simulink model "GhendyanoT2FMeioLinha1"  (R2021b)
settings: Solver=ode45  StartTime=0.0  StopTime=TempoSimulacao  RelTol=1e-3  EnableMultiTasking=on
values from neighbouring files (symbols this model uses):
  ccc1 = Ccc*d    [TesteRealCurtoFuses.m]    (also in TesteRealCurto_SemFuse.m)
  ccc2 = Ccc*d    [TesteRealCurtoFuses.m]    (also in TesteRealCurto_SemFuse.m)
  cct1 = Cct*d    [TesteRealCurtoFuses.m]    (also in TesteRealCurto_SemFuse.m)
  cct2 = Cct*d    [TesteRealCurtoFuses.m]    (also in TesteRealCurto_SemFuse.m)
  cequa1 = Ceq*d    [TesteRealCurtoFuses.m]    (also in TesteRealCurto_SemFuse.m)
  cequa2 = Ceq*d    [TesteRealCurtoFuses.m]    (also in TesteRealCurto_SemFuse.m)
  FatorSimulacao = 1e-3    (= 0.001)    [TesteRealCurtoFuses.m]    (also in TesteRealCurto_SemFuse.m)
  le = 1e-10    [TesteRealCurto.m]    (also in TesteRealCurtoFuses.m; TesteRealCurto_SemFuse.m)
  lm1 = lm    [TesteRealCurto.m]    (also in TesteRealCurtoFuses.m; TesteRealCurto_SemFuse.m)
  lm2 = lm    [TesteRealCurto.m]    (also in TesteRealCurtoFuses.m; TesteRealCurto_SemFuse.m)
  lp1 = lp    [TesteRealCurto.m]    (also in TesteRealCurtoFuses.m; TesteRealCurto_SemFuse.m)
  lp2 = lp    [TesteRealCurto.m]    (also in TesteRealCurtoFuses.m; TesteRealCurto_SemFuse.m)
  NRE = 1e-12    [TesteRealCurto.m]    (also in TesteRealCurtoFuses.m; TesteRealCurto_SemFuse.m)
  Raf1 = inf    [TesteRealCurto.m]    (also in TesteRealCurtoFuses.m; TesteRealCurto_SemFuse.m)
  Raf2 = inf    [TesteRealCurto.m]    (also in TesteRealCurtoFuses.m; TesteRealCurto_SemFuse.m)
  Rbf1 = inf    [TesteRealCurto.m]    (also in TesteRealCurtoFuses.m; TesteRealCurto_SemFuse.m)
  Rbf2 = inf    [TesteRealCurto.m]    (also in TesteRealCurtoFuses.m; TesteRealCurto_SemFuse.m)
  Rcf1 = inf    [TesteRealCurto.m]    (also in TesteRealCurtoFuses.m; TesteRealCurto_SemFuse.m)
  Rcf2 = inf    [TesteRealCurto.m]    (also in TesteRealCurtoFuses.m; TesteRealCurto_SemFuse.m)
  rm1 = rm    [TesteRealCurto.m]    (also in TesteRealCurtoFuses.m; TesteRealCurto_SemFuse.m)
  rm2 = rm    [TesteRealCurto.m]    (also in TesteRealCurtoFuses.m; TesteRealCurto_SemFuse.m)
  rp1 = rp    [TesteRealCurto.m]    (also in TesteRealCurtoFuses.m; TesteRealCurto_SemFuse.m)
  rp2 = rp    [TesteRealCurto.m]    (also in TesteRealCurtoFuses.m; TesteRealCurto_SemFuse.m)
  rtc1 = 8    [TesteRealCurto.m]    (also in TesteRealCurtoFuses.m; TesteRealCurto_SemFuse.m)
  rtc2 = 8    [TesteRealCurto.m]    (also in TesteRealCurtoFuses.m; TesteRealCurto_SemFuse.m)
  rti = 10    [TesteRealCurto.m]    (also in TesteRealCurtoFuses.m; TesteRealCurto_SemFuse.m)
undefined symbols (not defined in the file or in its folder): D11, Delta, m1
libraries: spsSeriesRLCBranchLib x26, spsRMSLib x14, spsBreakerLib x9, spsCurrentMeasurementLib x9, spsThreePhaseTransformerTwoWindingsLib x4, spsThreePhaseVIMeasurementLib x3, spsMutualInductanceLib x3, spsThreePhaseSeriesRLCLoadLib x2, spsThreePhaseSourceLib x1, spspowerguiLib x1
(part 2 of 2)

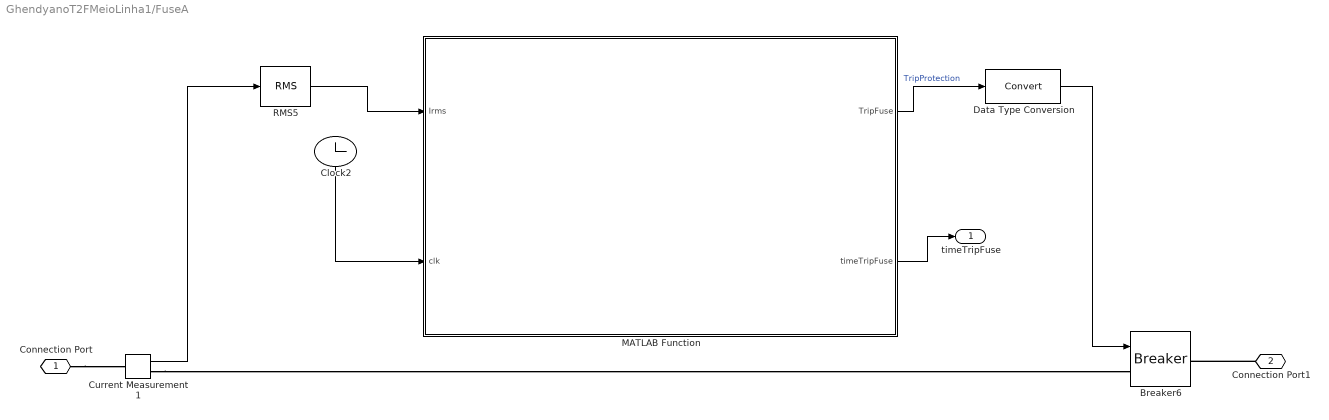
== system GhendyanoT2FMeioLinha1/FuseA ==
  Breaker6 : spsBreakerLib/Breaker  InitialState=1  SwitchingTimes="[1/60  5/60]"  External=on  BreakerResistance=0.01  SnubberResistance=1e6  SnubberCapacitance=inf  Measurements=None  MoreParameters=on  NoBreakLoop=off
      settings: SourceProductBaseCode=PS
  Clock2 : Clock
      settings: Decimation=1000
  Current Measurement1 : spsCurrentMeasurementLib/Current Measurement  PhasorSimulation=off  OutputType=Complex  PSBequivalent=0
  Data Type Conversion : DataTypeConversion
  MATLAB Function : MATLAB Function
  RMS5 : spsRMSLib/RMS  TrueRMS=on  Freq=60  RMSInit=0  Ts=0
  Connection Port : PMIOPort  Side=Right
  Connection Port1 : PMIOPort  Port=2  Side=Left
  timeTripFuse : Outport
  wires:
  MATLAB Function/1(TripFuse) -> Data Type Conversion/1  "TripProtection"
  RMS5/1 -> MATLAB Function/1(Irms)
  Data Type Conversion/1 -> Breaker6/1
  Current Measurement1/1 -> RMS5/1
  Clock2/1 -> MATLAB Function/2(clk)
  MATLAB Function/2(timeTripFuse) -> timeTripFuse/1
  connections:
  Current Measurement1/RConn1 -- Breaker6/LConn1
  Connection Port/RConn1 -- Current Measurement1/LConn1
  Connection Port1/RConn1 -- Breaker6/RConn1

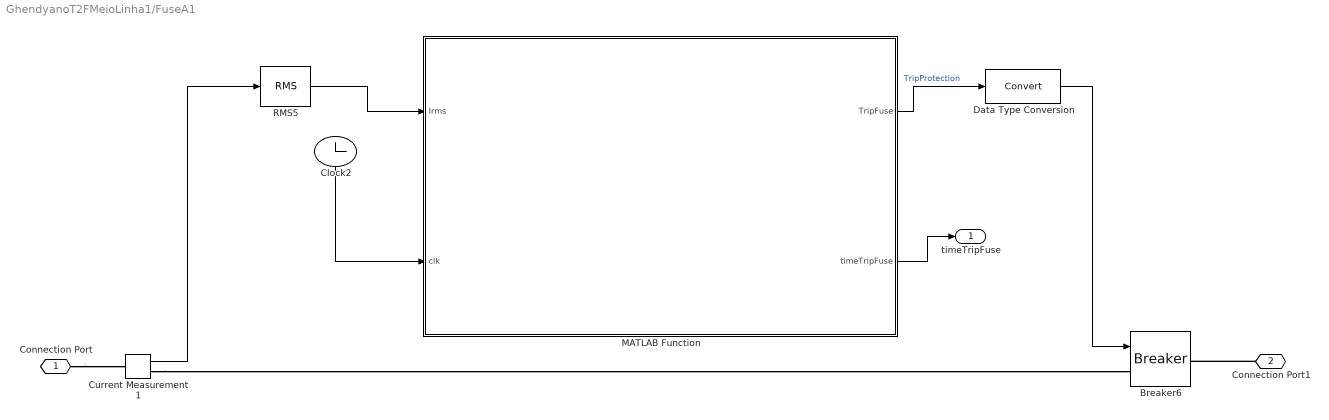
== system GhendyanoT2FMeioLinha1/FuseA1 ==
  Breaker6 : spsBreakerLib/Breaker  InitialState=1  SwitchingTimes="[1/60  5/60]"  External=on  BreakerResistance=0.01  SnubberResistance=1e6  SnubberCapacitance=inf  Measurements=None  MoreParameters=on  NoBreakLoop=off
      settings: SourceProductBaseCode=PS
  Clock2 : Clock
      settings: Decimation=1000
  Current Measurement1 : spsCurrentMeasurementLib/Current Measurement  PhasorSimulation=off  OutputType=Complex  PSBequivalent=0
  Data Type Conversion : DataTypeConversion
  MATLAB Function : MATLAB Function
  RMS5 : spsRMSLib/RMS  TrueRMS=on  Freq=60  RMSInit=0  Ts=0
  Connection Port : PMIOPort  Side=Right
  Connection Port1 : PMIOPort  Port=2  Side=Left
  timeTripFuse : Outport
  wires:
  MATLAB Function/1(TripFuse) -> Data Type Conversion/1  "TripProtection"
  RMS5/1 -> MATLAB Function/1(Irms)
  Data Type Conversion/1 -> Breaker6/1
  Current Measurement1/1 -> RMS5/1
  Clock2/1 -> MATLAB Function/2(clk)
  MATLAB Function/2(timeTripFuse) -> timeTripFuse/1
  connections:
  Current Measurement1/RConn1 -- Breaker6/LConn1
  Connection Port/RConn1 -- Current Measurement1/LConn1
  Connection Port1/RConn1 -- Breaker6/RConn1

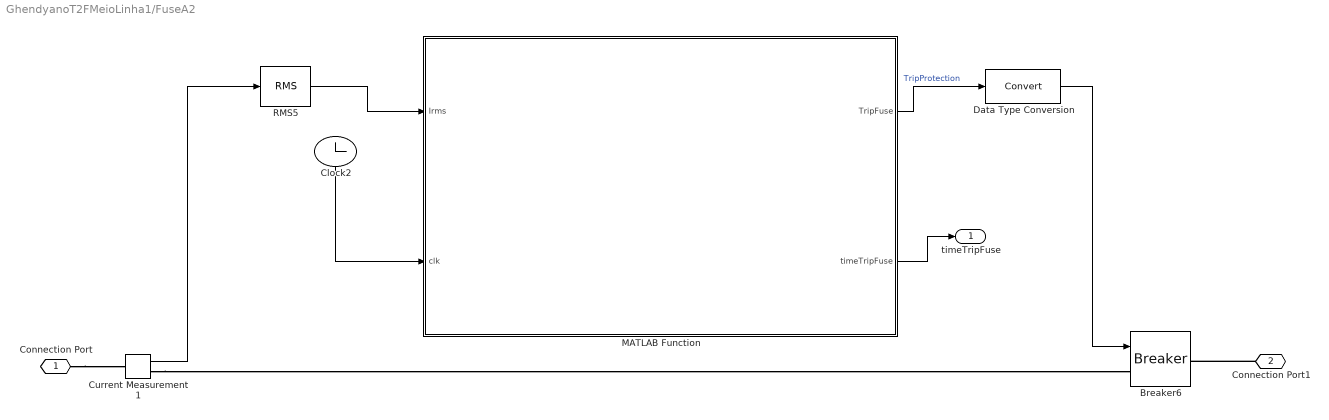
== system GhendyanoT2FMeioLinha1/FuseA2 ==
  Breaker6 : spsBreakerLib/Breaker  InitialState=1  SwitchingTimes="[1/60  5/60]"  External=on  BreakerResistance=0.01  SnubberResistance=1e6  SnubberCapacitance=inf  Measurements=None  MoreParameters=on  NoBreakLoop=off
      settings: SourceProductBaseCode=PS
  Clock2 : Clock
      settings: Decimation=1000
  Current Measurement1 : spsCurrentMeasurementLib/Current Measurement  PhasorSimulation=off  OutputType=Complex  PSBequivalent=0
  Data Type Conversion : DataTypeConversion
  MATLAB Function : MATLAB Function
  RMS5 : spsRMSLib/RMS  TrueRMS=on  Freq=60  RMSInit=0  Ts=0
  Connection Port : PMIOPort  Side=Right
  Connection Port1 : PMIOPort  Port=2  Side=Left
  timeTripFuse : Outport
  wires:
  MATLAB Function/1(TripFuse) -> Data Type Conversion/1  "TripProtection"
  RMS5/1 -> MATLAB Function/1(Irms)
  Data Type Conversion/1 -> Breaker6/1
  Current Measurement1/1 -> RMS5/1
  Clock2/1 -> MATLAB Function/2(clk)
  MATLAB Function/2(timeTripFuse) -> timeTripFuse/1
  connections:
  Current Measurement1/RConn1 -- Breaker6/LConn1
  Connection Port/RConn1 -- Current Measurement1/LConn1
  Connection Port1/RConn1 -- Breaker6/RConn1

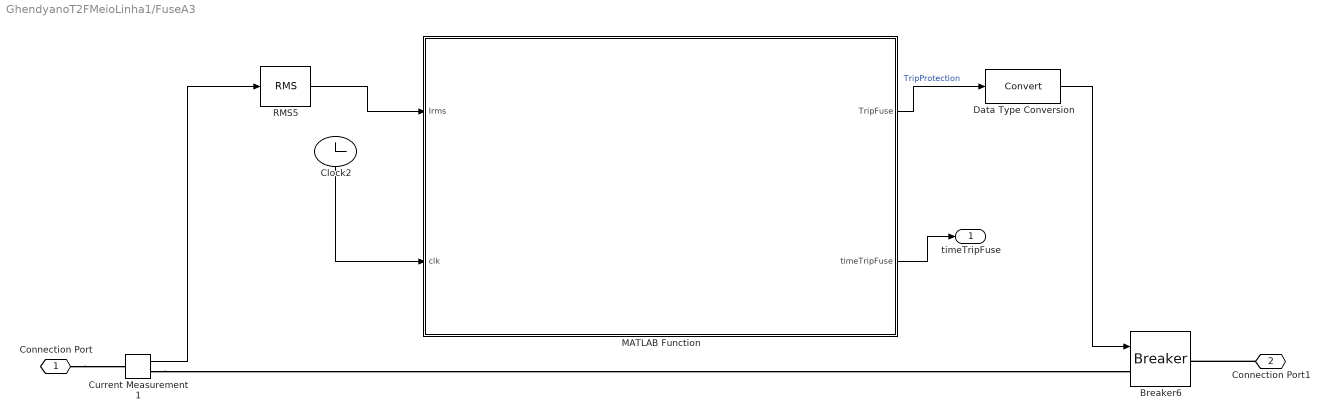
== system GhendyanoT2FMeioLinha1/FuseA3 ==
  Breaker6 : spsBreakerLib/Breaker  InitialState=1  SwitchingTimes="[1/60  5/60]"  External=on  BreakerResistance=0.01  SnubberResistance=1e6  SnubberCapacitance=inf  Measurements=None  MoreParameters=on  NoBreakLoop=off
      settings: SourceProductBaseCode=PS
  Clock2 : Clock
      settings: Decimation=1000
  Current Measurement1 : spsCurrentMeasurementLib/Current Measurement  PhasorSimulation=off  OutputType=Complex  PSBequivalent=0
  Data Type Conversion : DataTypeConversion
  MATLAB Function : MATLAB Function
  RMS5 : spsRMSLib/RMS  TrueRMS=on  Freq=60  RMSInit=0  Ts=0
  Connection Port : PMIOPort  Side=Right
  Connection Port1 : PMIOPort  Port=2  Side=Left
  timeTripFuse : Outport
  wires:
  MATLAB Function/1(TripFuse) -> Data Type Conversion/1  "TripProtection"
  RMS5/1 -> MATLAB Function/1(Irms)
  Data Type Conversion/1 -> Breaker6/1
  Current Measurement1/1 -> RMS5/1
  Clock2/1 -> MATLAB Function/2(clk)
  MATLAB Function/2(timeTripFuse) -> timeTripFuse/1
  connections:
  Current Measurement1/RConn1 -- Breaker6/LConn1
  Connection Port/RConn1 -- Current Measurement1/LConn1
  Connection Port1/RConn1 -- Breaker6/RConn1

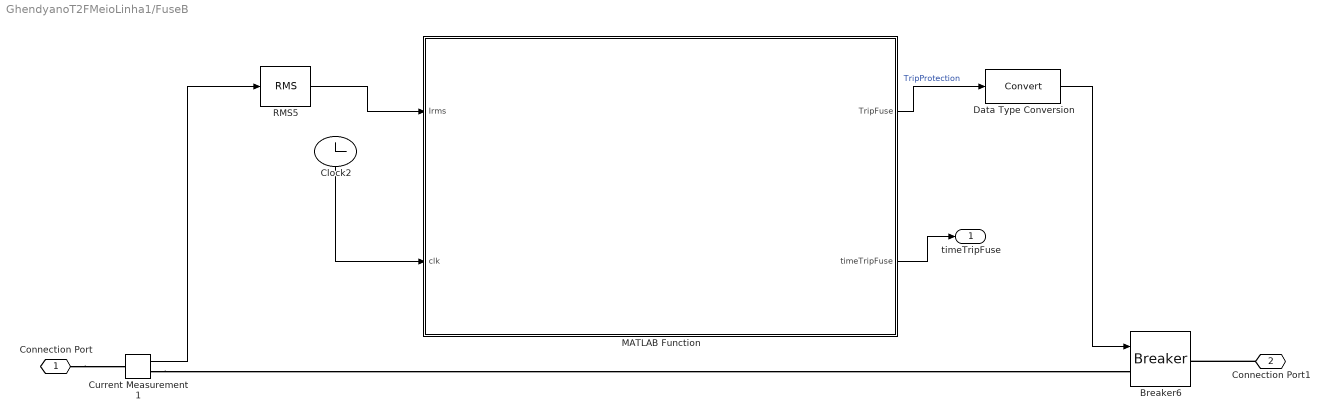
== system GhendyanoT2FMeioLinha1/FuseB ==
  Breaker6 : spsBreakerLib/Breaker  InitialState=1  SwitchingTimes="[1/60  5/60]"  External=on  BreakerResistance=0.01  SnubberResistance=1e6  SnubberCapacitance=inf  Measurements=None  MoreParameters=on  NoBreakLoop=off
      settings: SourceProductBaseCode=PS
  Clock2 : Clock
      settings: Decimation=1000
  Current Measurement1 : spsCurrentMeasurementLib/Current Measurement  PhasorSimulation=off  OutputType=Complex  PSBequivalent=0
  Data Type Conversion : DataTypeConversion
  MATLAB Function : MATLAB Function
  RMS5 : spsRMSLib/RMS  TrueRMS=on  Freq=60  RMSInit=0  Ts=0
  Connection Port : PMIOPort  Side=Right
  Connection Port1 : PMIOPort  Port=2  Side=Left
  timeTripFuse : Outport
  wires:
  MATLAB Function/1(TripFuse) -> Data Type Conversion/1  "TripProtection"
  RMS5/1 -> MATLAB Function/1(Irms)
  Data Type Conversion/1 -> Breaker6/1
  Current Measurement1/1 -> RMS5/1
  Clock2/1 -> MATLAB Function/2(clk)
  MATLAB Function/2(timeTripFuse) -> timeTripFuse/1
  connections:
  Current Measurement1/RConn1 -- Breaker6/LConn1
  Connection Port/RConn1 -- Current Measurement1/LConn1
  Connection Port1/RConn1 -- Breaker6/RConn1

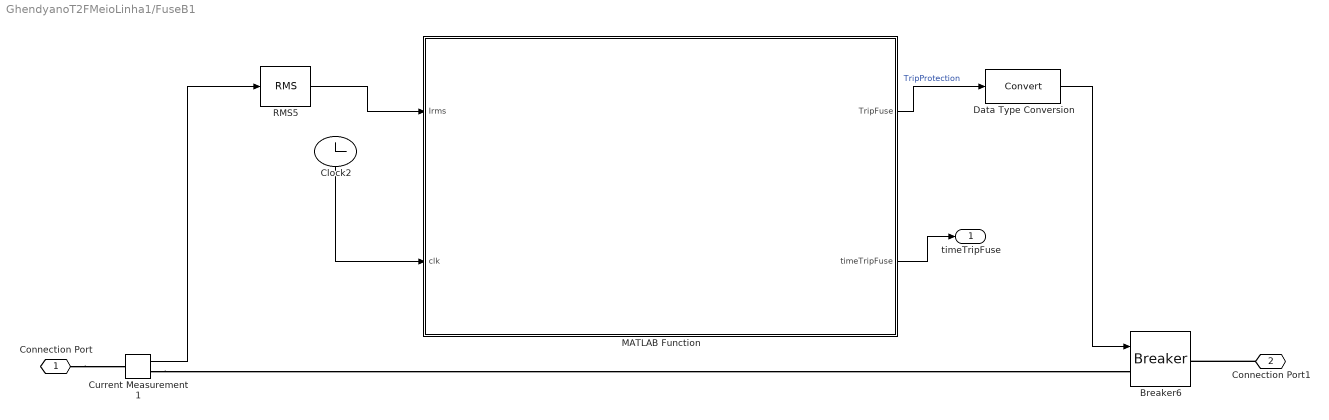
== system GhendyanoT2FMeioLinha1/FuseB1 ==
  Breaker6 : spsBreakerLib/Breaker  InitialState=1  SwitchingTimes="[1/60  5/60]"  External=on  BreakerResistance=0.01  SnubberResistance=1e6  SnubberCapacitance=inf  Measurements=None  MoreParameters=on  NoBreakLoop=off
      settings: SourceProductBaseCode=PS
  Clock2 : Clock
      settings: Decimation=1000
  Current Measurement1 : spsCurrentMeasurementLib/Current Measurement  PhasorSimulation=off  OutputType=Complex  PSBequivalent=0
  Data Type Conversion : DataTypeConversion
  MATLAB Function : MATLAB Function
  RMS5 : spsRMSLib/RMS  TrueRMS=on  Freq=60  RMSInit=0  Ts=0
  Connection Port : PMIOPort  Side=Right
  Connection Port1 : PMIOPort  Port=2  Side=Left
  timeTripFuse : Outport
  wires:
  MATLAB Function/1(TripFuse) -> Data Type Conversion/1  "TripProtection"
  RMS5/1 -> MATLAB Function/1(Irms)
  Data Type Conversion/1 -> Breaker6/1
  Current Measurement1/1 -> RMS5/1
  Clock2/1 -> MATLAB Function/2(clk)
  MATLAB Function/2(timeTripFuse) -> timeTripFuse/1
  connections:
  Current Measurement1/RConn1 -- Breaker6/LConn1
  Connection Port/RConn1 -- Current Measurement1/LConn1
  Connection Port1/RConn1 -- Breaker6/RConn1

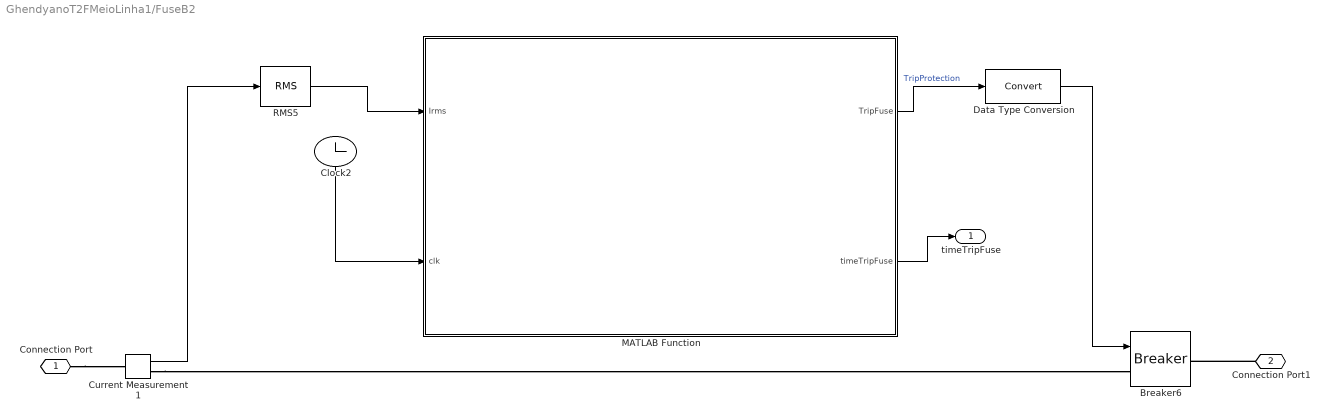
== system GhendyanoT2FMeioLinha1/FuseB2 ==
  Breaker6 : spsBreakerLib/Breaker  InitialState=1  SwitchingTimes="[1/60  5/60]"  External=on  BreakerResistance=0.01  SnubberResistance=1e6  SnubberCapacitance=inf  Measurements=None  MoreParameters=on  NoBreakLoop=off
      settings: SourceProductBaseCode=PS
  Clock2 : Clock
      settings: Decimation=1000
  Current Measurement1 : spsCurrentMeasurementLib/Current Measurement  PhasorSimulation=off  OutputType=Complex  PSBequivalent=0
  Data Type Conversion : DataTypeConversion
  MATLAB Function : MATLAB Function
  RMS5 : spsRMSLib/RMS  TrueRMS=on  Freq=60  RMSInit=0  Ts=0
  Connection Port : PMIOPort  Side=Right
  Connection Port1 : PMIOPort  Port=2  Side=Left
  timeTripFuse : Outport
  wires:
  MATLAB Function/1(TripFuse) -> Data Type Conversion/1  "TripProtection"
  RMS5/1 -> MATLAB Function/1(Irms)
  Data Type Conversion/1 -> Breaker6/1
  Current Measurement1/1 -> RMS5/1
  Clock2/1 -> MATLAB Function/2(clk)
  MATLAB Function/2(timeTripFuse) -> timeTripFuse/1
  connections:
  Current Measurement1/RConn1 -- Breaker6/LConn1
  Connection Port/RConn1 -- Current Measurement1/LConn1
  Connection Port1/RConn1 -- Breaker6/RConn1

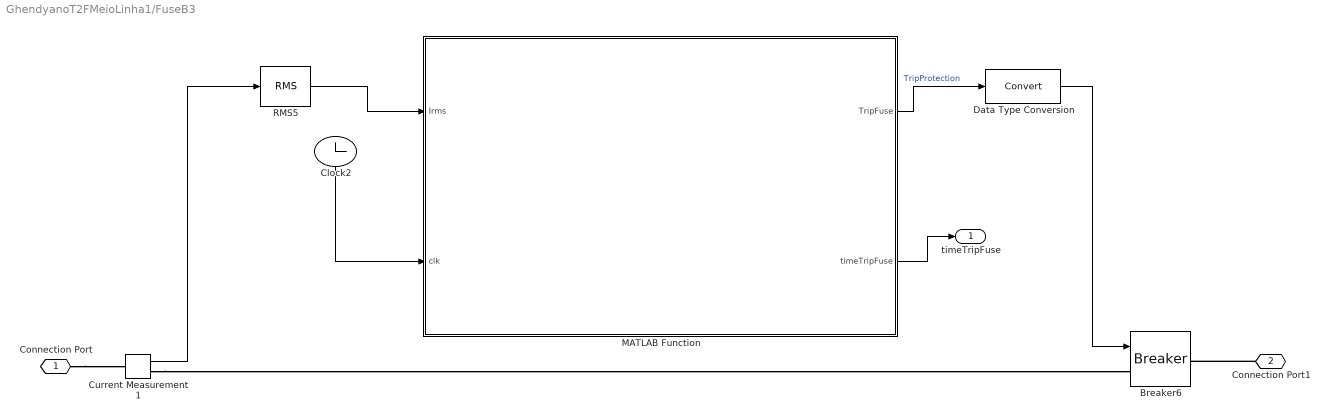
== system GhendyanoT2FMeioLinha1/FuseB3 ==
  Breaker6 : spsBreakerLib/Breaker  InitialState=1  SwitchingTimes="[1/60  5/60]"  External=on  BreakerResistance=0.01  SnubberResistance=1e6  SnubberCapacitance=inf  Measurements=None  MoreParameters=on  NoBreakLoop=off
      settings: SourceProductBaseCode=PS
  Clock2 : Clock
      settings: Decimation=1000
  Current Measurement1 : spsCurrentMeasurementLib/Current Measurement  PhasorSimulation=off  OutputType=Complex  PSBequivalent=0
  Data Type Conversion : DataTypeConversion
  MATLAB Function : MATLAB Function
  RMS5 : spsRMSLib/RMS  TrueRMS=on  Freq=60  RMSInit=0  Ts=0
  Connection Port : PMIOPort  Side=Right
  Connection Port1 : PMIOPort  Port=2  Side=Left
  timeTripFuse : Outport
  wires:
  MATLAB Function/1(TripFuse) -> Data Type Conversion/1  "TripProtection"
  RMS5/1 -> MATLAB Function/1(Irms)
  Data Type Conversion/1 -> Breaker6/1
  Current Measurement1/1 -> RMS5/1
  Clock2/1 -> MATLAB Function/2(clk)
  MATLAB Function/2(timeTripFuse) -> timeTripFuse/1
  connections:
  Current Measurement1/RConn1 -- Breaker6/LConn1
  Connection Port/RConn1 -- Current Measurement1/LConn1
  Connection Port1/RConn1 -- Breaker6/RConn1

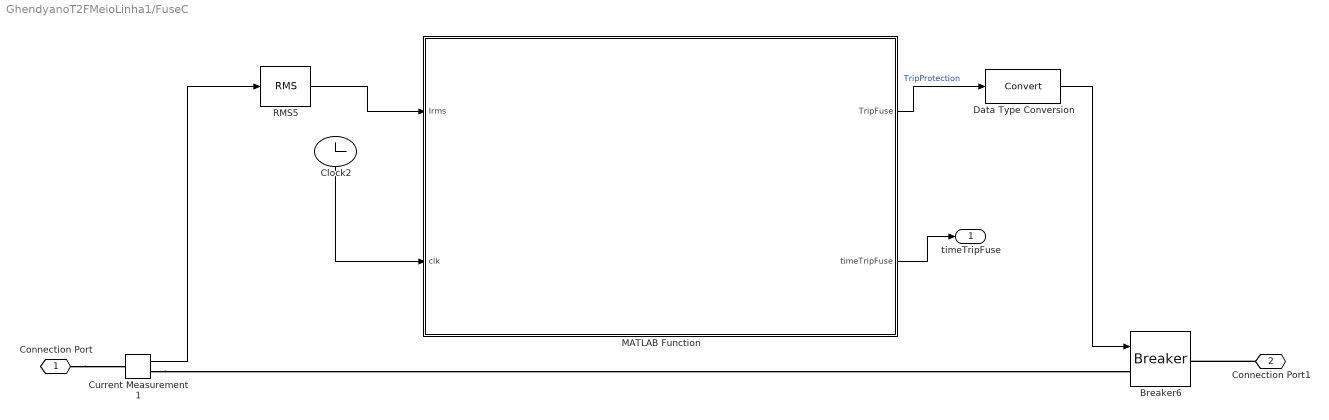
== system GhendyanoT2FMeioLinha1/FuseC ==
  Breaker6 : spsBreakerLib/Breaker  InitialState=1  SwitchingTimes="[1/60  5/60]"  External=on  BreakerResistance=0.01  SnubberResistance=1e6  SnubberCapacitance=inf  Measurements=None  MoreParameters=on  NoBreakLoop=off
      settings: SourceProductBaseCode=PS
  Clock2 : Clock
      settings: Decimation=1000
  Current Measurement1 : spsCurrentMeasurementLib/Current Measurement  PhasorSimulation=off  OutputType=Complex  PSBequivalent=0
  Data Type Conversion : DataTypeConversion
  MATLAB Function : MATLAB Function
  RMS5 : spsRMSLib/RMS  TrueRMS=on  Freq=60  RMSInit=0  Ts=0
  Connection Port : PMIOPort  Side=Right
  Connection Port1 : PMIOPort  Port=2  Side=Left
  timeTripFuse : Outport
  wires:
  MATLAB Function/1(TripFuse) -> Data Type Conversion/1  "TripProtection"
  RMS5/1 -> MATLAB Function/1(Irms)
  Data Type Conversion/1 -> Breaker6/1
  Current Measurement1/1 -> RMS5/1
  Clock2/1 -> MATLAB Function/2(clk)
  MATLAB Function/2(timeTripFuse) -> timeTripFuse/1
  connections:
  Current Measurement1/RConn1 -- Breaker6/LConn1
  Connection Port/RConn1 -- Current Measurement1/LConn1
  Connection Port1/RConn1 -- Breaker6/RConn1

== matlab function GhendyanoT2FMeioLinha1/FuseB1/MATLAB Function ==
  settings: updateMethod=DISCRETE
  data: Irms input; clk input; TripFuse output; a parameter; b parameter; c parameter; d parameter; e parameter; timeTripFuse output; IoTot parameter
function [TripFuse, timeTripFuse ]  =  fcn(Irms, clk, a, b, c, d, e, IoTot)
persistent RelayStateOvercurrentTime OperatingTime PickupTime TripTime signal valorIRMS y t timeTrip ValorAbertura
if isempty(RelayStateOvercurrentTime)
    RelayStateOvercurrentTime = 0;
    TripTime = 0;
    signal = 1;
    OperatingTime = inf;
    PickupTime = 0;
    valorIRMS = 0;
    timeTrip = inf;
    ValorAbertura = inf;
end

%% tripFuse
if (RelayStateOvercurrentTime == 0)&&(Irms > IoTot*3)
    PickupTime = clk+0.07;
    RelayStateOvercurrentTime = 1;
end

if(RelayStateOvercurrentTime == 1)&&(clk>PickupTime)
    valorIRMS = Irms;
    y = log(valorIRMS);
    t = a + (b * y) + (c * y^2) + (d * y^3) + (e * y^4);
    OperatingTime = exp(t);
    TripTime = PickupTime + OperatingTime;
    RelayStateOvercurrentTime = 2;
end

if (clk > TripTime)&&(RelayStateOvercurrentTime == 2)
    if ((Irms <= valorIRMS*0.5)&&(Irms <= IoTot*3))
        signal = 1;
        RelayStateOvercurrentTime = 0;
        TripTime = inf;
    else
        ValorAbertura = clk;
        signal = 0;
        RelayStateOvercurrentTime = 3;
        timeTrip = OperatingTime;
    end
end

TripFuse = signal;
timeTripFuse = [valorIRMS timeTrip ValorAbertura];

== matlab function GhendyanoT2FMeioLinha1/FuseA3/MATLAB Function ==
  settings: updateMethod=DISCRETE
  data: Irms input; clk input; TripFuse output; a parameter; b parameter; c parameter; d parameter; e parameter; timeTripFuse output; IoTot parameter
function [TripFuse, timeTripFuse ]  =  fcn(Irms, clk, a, b, c, d, e, IoTot)
persistent RelayStateOvercurrentTime OperatingTime PickupTime TripTime signal valorIRMS y t timeTrip ValorAbertura
if isempty(RelayStateOvercurrentTime)
    RelayStateOvercurrentTime = 0;
    TripTime = 0;
    signal = 1;
    OperatingTime = inf;
    PickupTime = 0;
    valorIRMS = 0;
    timeTrip = inf;
    ValorAbertura = inf;
end

%% tripFuse
if (RelayStateOvercurrentTime == 0)&&(Irms > IoTot*3)
    PickupTime = clk+0.07;
    RelayStateOvercurrentTime = 1;
end

if(RelayStateOvercurrentTime == 1)&&(clk>PickupTime)
    valorIRMS = Irms;
    y = log(valorIRMS);
    t = a + (b * y) + (c * y^2) + (d * y^3) + (e * y^4);
    OperatingTime = exp(t);
    TripTime = PickupTime + OperatingTime;
    RelayStateOvercurrentTime = 2;
end

if (clk > TripTime)&&(RelayStateOvercurrentTime == 2)
    if ((Irms <= valorIRMS*0.5)&&(Irms <= IoTot*3))
        signal = 1;
        RelayStateOvercurrentTime = 0;
        TripTime = inf;
    else
        ValorAbertura = clk;
        signal = 0;
        RelayStateOvercurrentTime = 3;
        timeTrip = OperatingTime;
    end
end

TripFuse = signal;
timeTripFuse = [valorIRMS timeTrip ValorAbertura];

== matlab function GhendyanoT2FMeioLinha1/FuseB3/MATLAB Function ==
  settings: updateMethod=DISCRETE
  data: Irms input; clk input; TripFuse output; a parameter; b parameter; c parameter; d parameter; e parameter; timeTripFuse output; IoTot parameter
function [TripFuse, timeTripFuse ]  =  fcn(Irms, clk, a, b, c, d, e, IoTot)
persistent RelayStateOvercurrentTime OperatingTime PickupTime TripTime signal valorIRMS y t timeTrip ValorAbertura
if isempty(RelayStateOvercurrentTime)
    RelayStateOvercurrentTime = 0;
    TripTime = 0;
    signal = 1;
    OperatingTime = inf;
    PickupTime = 0;
    valorIRMS = 0;
    timeTrip = inf;
    ValorAbertura = inf;
end

%% tripFuse
if (RelayStateOvercurrentTime == 0)&&(Irms > IoTot*3)
    PickupTime = clk+0.07;
    RelayStateOvercurrentTime = 1;
end

if(RelayStateOvercurrentTime == 1)&&(clk>PickupTime)
    valorIRMS = Irms;
    y = log(valorIRMS);
    t = a + (b * y) + (c * y^2) + (d * y^3) + (e * y^4);
    OperatingTime = exp(t);
    TripTime = PickupTime + OperatingTime;
    RelayStateOvercurrentTime = 2;
end

if (clk > TripTime)&&(RelayStateOvercurrentTime == 2)
    if ((Irms <= valorIRMS*0.5)&&(Irms <= IoTot*3))
        signal = 1;
        RelayStateOvercurrentTime = 0;
        TripTime = inf;
    else
        ValorAbertura = clk;
        signal = 0;
        RelayStateOvercurrentTime = 3;
        timeTrip = OperatingTime;
    end
end

TripFuse = signal;
timeTripFuse = [valorIRMS timeTrip ValorAbertura];

== matlab function GhendyanoT2FMeioLinha1/FuseA/MATLAB Function ==
  settings: updateMethod=DISCRETE
  data: Irms input; clk input; TripFuse output; a parameter; b parameter; c parameter; d parameter; e parameter; timeTripFuse output; IoTot parameter
function [TripFuse, timeTripFuse ]  =  fcn(Irms, clk, a, b, c, d, e, IoTot)
persistent RelayStateOvercurrentTime OperatingTime PickupTime TripTime signal valorIRMS y t timeTrip ValorAbertura
if isempty(RelayStateOvercurrentTime)
    RelayStateOvercurrentTime = 0;
    TripTime = 0;
    signal = 1;
    OperatingTime = inf;
    PickupTime = 0;
    valorIRMS = 0;
    timeTrip = inf;
    ValorAbertura = inf;
end

%% tripFuse
if (RelayStateOvercurrentTime == 0)&&(Irms > IoTot*3)
    PickupTime = clk+0.07;
    RelayStateOvercurrentTime = 1;
end

if(RelayStateOvercurrentTime == 1)&&(clk>PickupTime)
    valorIRMS = Irms;
    y = log(valorIRMS);
    t = a + (b * y) + (c * y^2) + (d * y^3) + (e * y^4);
    OperatingTime = exp(t);
    TripTime = PickupTime + OperatingTime;
    RelayStateOvercurrentTime = 2;
end

if (clk > TripTime)&&(RelayStateOvercurrentTime == 2)
    if ((Irms <= valorIRMS*0.5)&&(Irms <= IoTot*3))
        signal = 1;
        RelayStateOvercurrentTime = 0;
        TripTime = inf;
    else
        ValorAbertura = clk;
        signal = 0;
        RelayStateOvercurrentTime = 3;
        timeTrip = OperatingTime;
    end
end

TripFuse = signal;
timeTripFuse = [valorIRMS timeTrip ValorAbertura];

== matlab function GhendyanoT2FMeioLinha1/FuseB/MATLAB Function ==
  settings: updateMethod=DISCRETE
  data: Irms input; clk input; TripFuse output; a parameter; b parameter; c parameter; d parameter; e parameter; timeTripFuse output; IoTot parameter
function [TripFuse, timeTripFuse ]  =  fcn(Irms, clk, a, b, c, d, e, IoTot)
persistent RelayStateOvercurrentTime OperatingTime PickupTime TripTime signal valorIRMS y t timeTrip ValorAbertura
if isempty(RelayStateOvercurrentTime)
    RelayStateOvercurrentTime = 0;
    TripTime = 0;
    signal = 1;
    OperatingTime = inf;
    PickupTime = 0;
    valorIRMS = 0;
    timeTrip = inf;
    ValorAbertura = inf;
end

%% tripFuse
if (RelayStateOvercurrentTime == 0)&&(Irms > IoTot*3)
    PickupTime = clk+0.07;
    RelayStateOvercurrentTime = 1;
end

if(RelayStateOvercurrentTime == 1)&&(clk>PickupTime)
    valorIRMS = Irms;
    y = log(valorIRMS);
    t = a + (b * y) + (c * y^2) + (d * y^3) + (e * y^4);
    OperatingTime = exp(t);
    TripTime = PickupTime + OperatingTime;
    RelayStateOvercurrentTime = 2;
end

if (clk > TripTime)&&(RelayStateOvercurrentTime == 2)
    if ((Irms <= valorIRMS*0.5)&&(Irms <= IoTot*3))
        signal = 1;
        RelayStateOvercurrentTime = 0;
        TripTime = inf;
    else
        ValorAbertura = clk;
        signal = 0;
        RelayStateOvercurrentTime = 3;
        timeTrip = OperatingTime;
    end
end

TripFuse = signal;
timeTripFuse = [valorIRMS timeTrip ValorAbertura];

== matlab function GhendyanoT2FMeioLinha1/FuseC/MATLAB Function ==
  settings: updateMethod=DISCRETE
  data: Irms input; clk input; TripFuse output; a parameter; b parameter; c parameter; d parameter; e parameter; timeTripFuse output; IoTot parameter
function [TripFuse, timeTripFuse ]  =  fcn(Irms, clk, a, b, c, d, e, IoTot)
persistent RelayStateOvercurrentTime OperatingTime PickupTime TripTime signal valorIRMS y t timeTrip ValorAbertura
if isempty(RelayStateOvercurrentTime)
    RelayStateOvercurrentTime = 0;
    TripTime = 0;
    signal = 1;
    OperatingTime = inf;
    PickupTime = 0;
    valorIRMS = 0;
    timeTrip = inf;
    ValorAbertura = inf;
end

%% tripFuse
if (RelayStateOvercurrentTime == 0)&&(Irms > IoTot*3)
    PickupTime = clk+0.07;
    RelayStateOvercurrentTime = 1;
end

if(RelayStateOvercurrentTime == 1)&&(clk>PickupTime)
    valorIRMS = Irms;
    y = log(valorIRMS);
    t = a + (b * y) + (c * y^2) + (d * y^3) + (e * y^4);
    OperatingTime = exp(t);
    TripTime = PickupTime + OperatingTime;
    RelayStateOvercurrentTime = 2;
end

if (clk > TripTime)&&(RelayStateOvercurrentTime == 2)
    if ((Irms <= valorIRMS*0.5)&&(Irms <= IoTot*3))
        signal = 1;
        RelayStateOvercurrentTime = 0;
        TripTime = inf;
    else
        ValorAbertura = clk;
        signal = 0;
        RelayStateOvercurrentTime = 3;
        timeTrip = OperatingTime;
    end
end

TripFuse = signal;
timeTripFuse = [valorIRMS timeTrip ValorAbertura];

== matlab function GhendyanoT2FMeioLinha1/FuseA2/MATLAB Function ==
  settings: updateMethod=DISCRETE
  data: Irms input; clk input; TripFuse output; a parameter; b parameter; c parameter; d parameter; e parameter; timeTripFuse output; IoTot parameter
function [TripFuse, timeTripFuse ]  =  fcn(Irms, clk, a, b, c, d, e, IoTot)
persistent RelayStateOvercurrentTime OperatingTime PickupTime TripTime signal valorIRMS y t timeTrip ValorAbertura
if isempty(RelayStateOvercurrentTime)
    RelayStateOvercurrentTime = 0;
    TripTime = 0;
    signal = 1;
    OperatingTime = inf;
    PickupTime = 0;
    valorIRMS = 0;
    timeTrip = inf;
    ValorAbertura = inf;
end

%% tripFuse
if (RelayStateOvercurrentTime == 0)&&(Irms > IoTot*3)
    PickupTime = clk+0.07;
    RelayStateOvercurrentTime = 1;
end

if(RelayStateOvercurrentTime == 1)&&(clk>PickupTime)
    valorIRMS = Irms;
    y = log(valorIRMS);
    t = a + (b * y) + (c * y^2) + (d * y^3) + (e * y^4);
    OperatingTime = exp(t);
    TripTime = PickupTime + OperatingTime;
    RelayStateOvercurrentTime = 2;
end

if (clk > TripTime)&&(RelayStateOvercurrentTime == 2)
    if ((Irms <= valorIRMS*0.5)&&(Irms <= IoTot*3))
        signal = 1;
        RelayStateOvercurrentTime = 0;
        TripTime = inf;
    else
        ValorAbertura = clk;
        signal = 0;
        RelayStateOvercurrentTime = 3;
        timeTrip = OperatingTime;
    end
end

TripFuse = signal;
timeTripFuse = [valorIRMS timeTrip ValorAbertura];

== matlab function GhendyanoT2FMeioLinha1/FuseB2/MATLAB Function ==
  settings: updateMethod=DISCRETE
  data: Irms input; clk input; TripFuse output; a parameter; b parameter; c parameter; d parameter; e parameter; timeTripFuse output; IoTot parameter
function [TripFuse, timeTripFuse ]  =  fcn(Irms, clk, a, b, c, d, e, IoTot)
persistent RelayStateOvercurrentTime OperatingTime PickupTime TripTime signal valorIRMS y t timeTrip ValorAbertura
if isempty(RelayStateOvercurrentTime)
    RelayStateOvercurrentTime = 0;
    TripTime = 0;
    signal = 1;
    OperatingTime = inf;
    PickupTime = 0;
    valorIRMS = 0;
    timeTrip = inf;
    ValorAbertura = inf;
end

%% tripFuse
if (RelayStateOvercurrentTime == 0)&&(Irms > IoTot*3)
    PickupTime = clk+0.07;
    RelayStateOvercurrentTime = 1;
end

if(RelayStateOvercurrentTime == 1)&&(clk>PickupTime)
    valorIRMS = Irms;
    y = log(valorIRMS);
    t = a + (b * y) + (c * y^2) + (d * y^3) + (e * y^4);
    OperatingTime = exp(t);
    TripTime = PickupTime + OperatingTime;
    RelayStateOvercurrentTime = 2;
end

if (clk > TripTime)&&(RelayStateOvercurrentTime == 2)
    if ((Irms <= valorIRMS*0.5)&&(Irms <= IoTot*3))
        signal = 1;
        RelayStateOvercurrentTime = 0;
        TripTime = inf;
    else
        ValorAbertura = clk;
        signal = 0;
        RelayStateOvercurrentTime = 3;
        timeTrip = OperatingTime;
    end
end

TripFuse = signal;
timeTripFuse = [valorIRMS timeTrip ValorAbertura];

== matlab function GhendyanoT2FMeioLinha1/FuseA1/MATLAB Function ==
  settings: updateMethod=DISCRETE
  data: Irms input; clk input; TripFuse output; a parameter; b parameter; c parameter; d parameter; e parameter; timeTripFuse output; IoTot parameter
function [TripFuse, timeTripFuse ]  =  fcn(Irms, clk, a, b, c, d, e, IoTot)
persistent RelayStateOvercurrentTime OperatingTime PickupTime TripTime signal valorIRMS y t timeTrip ValorAbertura
if isempty(RelayStateOvercurrentTime)
    RelayStateOvercurrentTime = 0;
    TripTime = 0;
    signal = 1;
    OperatingTime = inf;
    PickupTime = 0;
    valorIRMS = 0;
    timeTrip = inf;
    ValorAbertura = inf;
end

%% tripFuse
if (RelayStateOvercurrentTime == 0)&&(Irms > IoTot*3)
    PickupTime = clk+0.07;
    RelayStateOvercurrentTime = 1;
end

if(RelayStateOvercurrentTime == 1)&&(clk>PickupTime)
    valorIRMS = Irms;
    y = log(valorIRMS);
    t = a + (b * y) + (c * y^2) + (d * y^3) + (e * y^4);
    OperatingTime = exp(t);
    TripTime = PickupTime + OperatingTime;
    RelayStateOvercurrentTime = 2;
end

if (clk > TripTime)&&(RelayStateOvercurrentTime == 2)
    if ((Irms <= valorIRMS*0.5)&&(Irms <= IoTot*3))
        signal = 1;
        RelayStateOvercurrentTime = 0;
        TripTime = inf;
    else
        ValorAbertura = clk;
        signal = 0;
        RelayStateOvercurrentTime = 3;
        timeTrip = OperatingTime;
    end
end

TripFuse = signal;
timeTripFuse = [valorIRMS timeTrip ValorAbertura];
